simulink model "is95revchtransmitter2"  (Simulink 4.00)
settings: Solver=VariableStepDiscrete  SolverMode=SingleTasking  StartTime=0.0  StopTime=0.1  RelTol=1e-3  AbsTol=1e-6
undefined symbols (not defined in the file or in its folder): slcm
libraries: cdmalibv1p1 x6, dspsigops x3, cdmaprivate x3, dspbuff3 x1
settings Model: CovMetricSettings=d  Creator=rkumar  LastModifiedBy=akansal  SaveTime=off  SaveOutput=off  LimitDataPoints=off  ExtModeTrigMode=oneshot  ExtModeArmWhenConnect=off  BlockReductionOpt=off

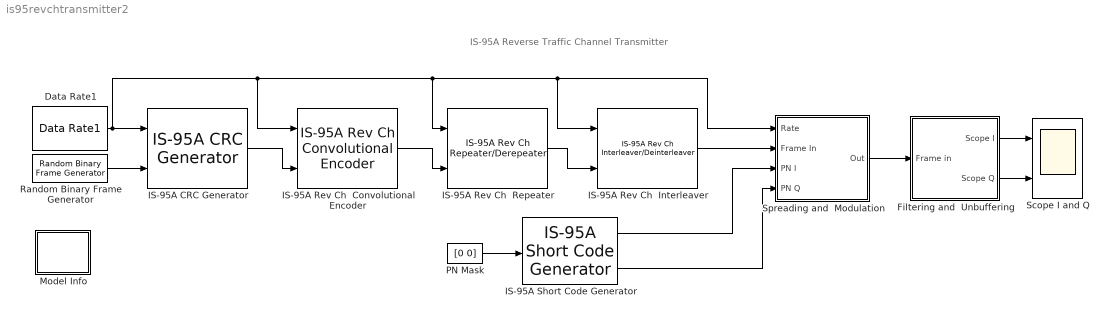
== system is95revchtransmitter2 ==
  note: IS-95A Reverse Traffic Channel Transmitter
  " Spreading and  Modulation" : Subsystem
      settings: RTWFcnNameOpts=Auto  RTWFileNameOpts=Auto
  Data Rate1 : cdmaprivate/Data Rate1  rate=Full
  "Filtering and  Unbuffering " : Subsystem
      settings: RTWFcnNameOpts=Auto  RTWFileNameOpts=Auto
  IS-95A CRC Generator : cdmalibv1p1/IS-95A Common/IS-95A CRC Generator  rate_set=Rate Set I  ch_type=Traffic
  IS-95A Rev Ch  Convolutional Encoder : cdmalibv1p1/IS-95A Mobile Station Transmitter/IS-95A Rev Ch Convolutional Encoder  rate_set=Rate Set I  ch_type=Traffic  enc_state=[]
  IS-95A Rev Ch  Interleaver : cdmalibv1p1/IS-95A Mobile Station Transmitter/IS-95A Rev Ch Interleaver//Deinterleaver  ch_type=Traffic  int_select=Interleaver
  IS-95A Rev Ch  Repeater : cdmalibv1p1/IS-95A Mobile Station Transmitter/IS-95A Rev Ch Repeater//Derepeater  ch_type=Traffic  rep_select=Derepeater
  IS-95A Short Code Generator : cdmalibv1p1/IS-95A Common/IS-95A Short Code Generator  numOut=64  sampTime=1/(50*384)
  Model Info : Subsystem  LoadFcn=slcm LoadBlock;  InitFcn=slcm('UpdateAllCMBlocksInThisModelInit')  mask(CMBlock){InitialSaveTempField=, InitialBlockCM=none, BlockCM=none, Frame=on, SaveTempField=, DisplayStringWithTags=Info, MaskDisplayString=Info, HorizontalTextAlignment=Center, LeftAlignmentValue=0.5, SourceBlockDiagram=is95revchtransmitter2, TagMaxNumber=20, CMTag1=, CMTag2=, CMTag3=, CMTag4=, CMTag5=, CMTag6=, CMTag7=, CMTag8=, CMTag9=, CMTag10=, CMTag11=, CMTag12=, CMTag13=, CMTag14=, CMTag15=, CMTag16=, CMTag17=, CMTag18=, CMTag19=, CMTag20=}
      mask help: This block allows revision control information to be displayed within the model.
      settings: CopyFcn=slcm CopyBlock;  DeleteFcn=slcm Cancel;  PostSaveFcn=slcm('UpdateAllCMBlocksInThisModel')  NameChangeFcn=slcm Rename;  OpenFcn=cdmademohelp;  RTWFcnNameOpts=Auto  RTWFileNameOpts=Auto
      mask Display: text(str2num(LeftAlignmentValue), 0.5, MaskDisplayString, 'HorizontalAlignment', HorizontalTextAlignment)
  PN Mask : Constant  Value=[0 0]
  Random Binary Frame Generator : cdmaprivate/Random Binary Frame Generator  seed=119940  Ts=1/(50*268)  N=268
  Scope I and Q : Scope  NumInputPorts=2
      settings: TickLabels=on  TimeRange=0.0001  YMin=-2~-2  YMax=2~2  SaveToWorkspace=off  SaveName=ScopeData  DataFormat=Array  LimitDataPoints=on  MaxDataPoints=5000
  wires:
  IS-95A Rev Ch  Convolutional Encoder/1 -> IS-95A Rev Ch  Repeater/2
  IS-95A CRC Generator/1 -> IS-95A Rev Ch  Convolutional Encoder/2
  IS-95A Rev Ch  Repeater/1 -> IS-95A Rev Ch  Interleaver/2
  IS-95A Rev Ch  Interleaver/1 -> " Spreading and  Modulation"/2(Frame In)
  PN Mask/1 -> IS-95A Short Code Generator/1
  IS-95A Short Code Generator/1 -> " Spreading and  Modulation"/3(PN I)
  "Filtering and  Unbuffering "/1(Scope I) -> Scope I and Q/1
  "Filtering and  Unbuffering "/2(Scope Q) -> Scope I and Q/2
  Random Binary Frame Generator/1 -> IS-95A CRC Generator/2
  Data Rate1/1 -> IS-95A Rev Ch  Convolutional Encoder/1, IS-95A Rev Ch  Repeater/1, IS-95A Rev Ch  Interleaver/1, " Spreading and  Modulation"/1(Rate), IS-95A CRC Generator/1
  " Spreading and  Modulation"/1("Out ") -> "Filtering and  Unbuffering "/1(Frame in)
  IS-95A Short Code Generator/2 -> " Spreading and  Modulation"/4(PN Q)

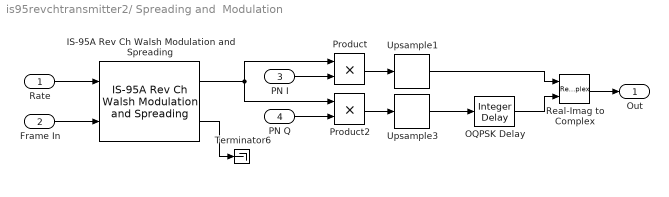
== system is95revchtransmitter2/ Spreading and  Modulation ==
  Rate : Inport  Port=1
  Frame In : Inport  Port=2
  PN I : Inport  Port=3
  PN Q : Inport  Port=4
  IS-95A Rev Ch Walsh Modulation and Spreading : cdmalibv1p1/IS-95A Mobile Station Transmitter/IS-95A Rev Ch Walsh Modulation and Spreading  chType=Traffic  lngCdMask=1  wlshOrd=6  sampTime=1/(50*384)
  OQPSK Delay : dspsigops/Integer Delay  delay=4  ic=0
  Product : Product  Inputs=2  Multiplication=Element-wise(.*)  SaturateOnIntegerOverflow=on
  Product2 : Product  Inputs=2  Multiplication=Element-wise(.*)  SaturateOnIntegerOverflow=on
  Real-Imag to Complex : RealImagToComplex  Input=RealAndImag  ConstantPart=0
  Terminator6 : Terminator
  Upsample1 : dspsigops/Upsample  N=8  phase=0  ic=0  mode=Maintain input frame rate
  Upsample3 : dspsigops/Upsample  N=8  phase=0  ic=0  mode=Maintain input frame rate
  "Out " : Outport  Port=1
  wires:
  Real-Imag to Complex/1 -> "Out "/1
  Upsample1/1 -> Real-Imag to Complex/1
  OQPSK Delay/1 -> Real-Imag to Complex/2
  Upsample3/1 -> OQPSK Delay/1
  Product2/1 -> Upsample3/1
  Product/1 -> Upsample1/1
  PN Q/1 -> Product2/2
  Frame In/1 -> IS-95A Rev Ch Walsh Modulation and Spreading/2
  IS-95A Rev Ch Walsh Modulation and Spreading/2 -> Terminator6/1
  PN I/1 -> Product/2
  Rate/1 -> IS-95A Rev Ch Walsh Modulation and Spreading/1
  IS-95A Rev Ch Walsh Modulation and Spreading/1 -> Product2/1, Product/1

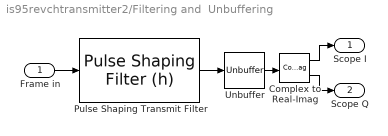
== system is95revchtransmitter2/Filtering and  Unbuffering  ==
  Frame in : Inport  Port=1
  Complex to Real-Imag : ComplexToRealImag  Output=RealAndImag
  Pulse Shaping Transmit Filter : cdmaprivate/Pulse Shaping Filter (h)  N=1
  Unbuffer : dspbuff3/Unbuffer  ic=0
  Scope I : Outport  Port=1
  Scope Q : Outport  Port=2
  wires:
  Frame in/1 -> Pulse Shaping Transmit Filter/1
  Pulse Shaping Transmit Filter/1 -> Unbuffer/1
  Unbuffer/1 -> Complex to Real-Imag/1
  Complex to Real-Imag/1 -> Scope I/1
  Complex to Real-Imag/2 -> Scope Q/1

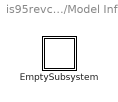
== system is95revchtransmitter2/Model Info ==
  EmptySubsystem : Subsystem
      settings: RTWFcnNameOpts=Auto  RTWFileNameOpts=Auto

== system is95revchtransmitter2/Model Info/EmptySubsystem ==
